simulink model "TKO_TA_KEL_10"  (R2021a)
settings: Solver=VariableStepAuto  StartTime=0.0  StopTime=10.0  RelTol=1e-3
settings Model: Creator=asus  LastModifiedBy=asus

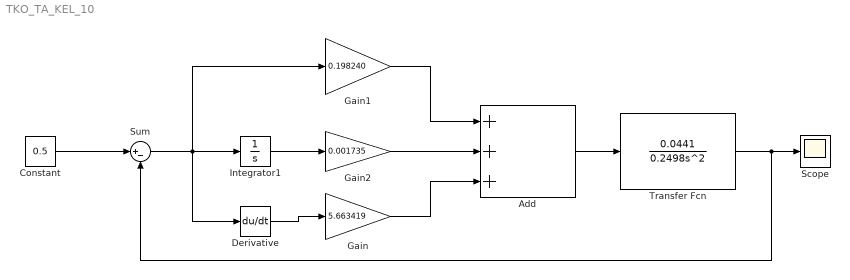
== system TKO_TA_KEL_10 ==
  Add : Sum  Inputs=+++
  Constant : Constant  Value=0.5
  Derivative : Derivative
  Gain : Gain  Gain=5.663419
  Gain1 : Gain  Gain=0.198240
  Gain2 : Gain  Gain=0.001735
  Integrator1 : Integrator
  Scope : Scope
  Sum : Sum  Inputs=|+-
  Transfer Fcn : TransferFcn  Numerator=[0.0441]  Denominator=[0.2498 0 0]
  wires:
  Constant/1 -> Sum/1
  Sum/1 -> Derivative/1, Gain1/1, Integrator1/1
  Integrator1/1 -> Gain2/1
  Derivative/1 -> Gain/1
  Gain1/1 -> Add/1
  Gain/1 -> Add/3
  Gain2/1 -> Add/2
  Add/1 -> Transfer Fcn/1
  Transfer Fcn/1 -> Sum/2, Scope/1
